simulink model "Buck_PI_DIGITAL_MG"  (R2024a)
settings: Solver=VariableStepAuto  StartTime=0.0  StopTime=0.1  RelTol=1e-3
libraries: spsSeriesRLCBranchLib x6, spsMeanLib x6, spsCurrentMeasurementLib x3, spsVoltageMeasurementLib x3, spsDiodeLib x2, spsDCVoltageSourceLib x2, spsMosfetLib x2, spsPWMGeneratorDCDCLib x2, sps_lib x1
settings Model: Creator=hardy  LastModifiedBy=marco
settings SolverCC: AlgebraicLoopSolver=TrustRegion
settings DebuggingCC: UnconnectedInputMsg=warning  UnconnectedOutputMsg=warning  UnconnectedLineMsg=warning
settings ModelReferenceCC: EnableRefExpFcnMdlSchedulingChecks=on
settings RTWCC: GPUComputeCapability=3.5

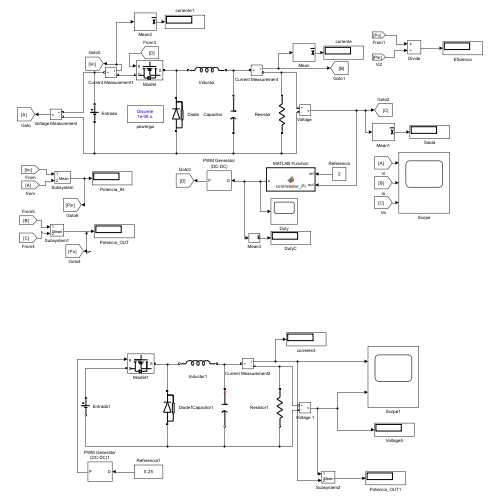
[thumbnail: Simulink's stored preview of the top-level diagram]
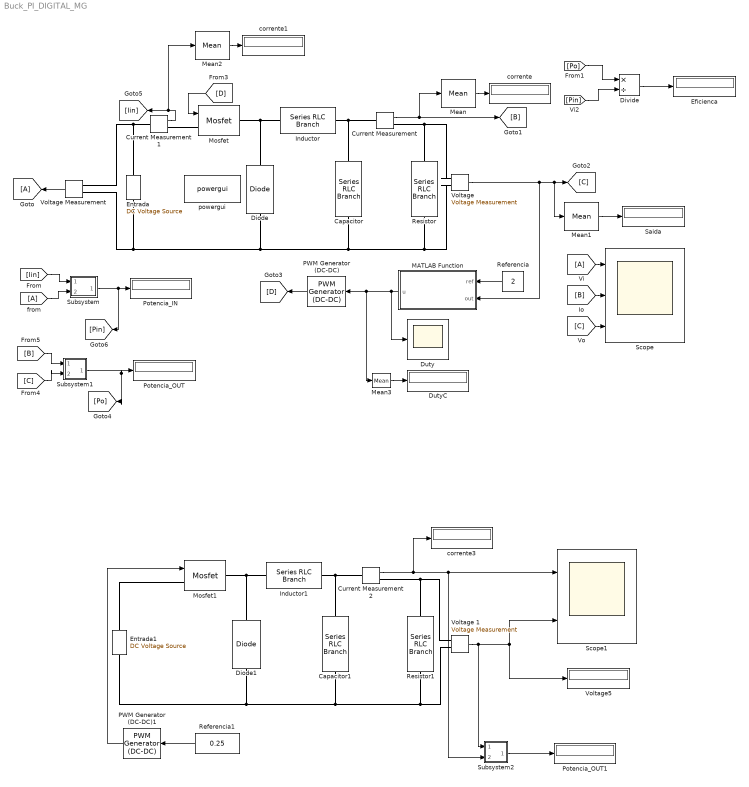
== system Buck_PI_DIGITAL_MG ==
  Capacitor : spsSeriesRLCBranchLib/Series RLC Branch  LConnTagsString=__new0  RConnTagsString=__new0  BranchType=C  Resistance=1  Inductance=1e-3  SetiL0=off  InitialCurrent=0  Capacitance=150e-6  Setx0=off  InitialVoltage=0  Measurements=None
  Capacitor1 : spsSeriesRLCBranchLib/Series RLC Branch  LConnTagsString=__new0  RConnTagsString=__new0  BranchType=C  Resistance=1  Inductance=1e-3  SetiL0=off  InitialCurrent=0  Capacitance=150e-6  Setx0=off  InitialVoltage=0  Measurements=None
  Current Measurement : spsCurrentMeasurementLib/Current Measurement  PhasorSimulation=off  OutputType=Complex  PSBequivalent=0
  Current Measurement1 : spsCurrentMeasurementLib/Current Measurement  PhasorSimulation=off  OutputType=Complex  PSBequivalent=0
  Current Measurement2 : spsCurrentMeasurementLib/Current Measurement  PhasorSimulation=off  OutputType=Complex  PSBequivalent=0
  Diode : spsDiodeLib/Diode  Ron=0.001  Lon=0  Vf=0  IC=0  UseSnubber=0  Rs=500  Cs=250e-9  Measurements=off
  Diode1 : spsDiodeLib/Diode  Ron=0.001  Lon=0  Vf=0  IC=0  UseSnubber=0  Rs=500  Cs=250e-9  Measurements=off
  Divide : Product  Inputs=*/
  Duty : Scope
  DutyC : Display
  Eficienca : Display
  Entrada : spsDCVoltageSourceLib/DC Voltage Source  Amplitude=10  Measurements=None
  Entrada1 : spsDCVoltageSourceLib/DC Voltage Source  Amplitude=10  Measurements=None
  Goto : Goto
  Inductor : spsSeriesRLCBranchLib/Series RLC Branch  LConnTagsString=__new0  RConnTagsString=__new0  BranchType=L  Resistance=1  Inductance=470e-6  SetiL0=off  InitialCurrent=0  Capacitance=1e-6  Setx0=off  InitialVoltage=0  Measurements=None
  Inductor1 : spsSeriesRLCBranchLib/Series RLC Branch  LConnTagsString=__new0  RConnTagsString=__new0  BranchType=L  Resistance=1  Inductance=470e-6  SetiL0=off  InitialCurrent=0  Capacitance=1e-6  Setx0=off  InitialVoltage=0  Measurements=None
  MATLAB Function : MATLAB Function  TreatAsAtomicUnit=on
  Mean{,1..3} (4 alike) : spsMeanLib/Mean  Freq=60  Vinit=0  Ts=0
  Mosfet : spsMosfetLib/Mosfet  Ron=0.1  Lon=0  Rd=0.01  Vfd=0  IC=0  Rs=1e5  Cs=inf  Measurements=off
  Mosfet1 : spsMosfetLib/Mosfet  Ron=0.1  Lon=0  Rd=0.01  Vfd=0  IC=0  Rs=1e5  Cs=inf  Measurements=off
  PWM Generator (DC-DC) : spsPWMGeneratorDCDCLib/PWM Generator (DC-DC)  Fsw=60000  Ts=1e-6
  PWM Generator (DC-DC)1 : spsPWMGeneratorDCDCLib/PWM Generator (DC-DC)  Fsw=60000  Ts=1e-6
  Potencia_IN : Display
  Potencia_OUT : Display
  Potencia_OUT1 : Display
  Referencia : Constant  Value=2
  Referencia1 : Constant  Value=0.25
  Resistor : spsSeriesRLCBranchLib/Series RLC Branch  LConnTagsString=__new0  RConnTagsString=__new0  BranchType=R  Resistance=1  Inductance=1e-3  SetiL0=off  InitialCurrent=0  Capacitance=1e-6  Setx0=off  InitialVoltage=0  Measurements=None
  Resistor1 : spsSeriesRLCBranchLib/Series RLC Branch  LConnTagsString=__new0  RConnTagsString=__new0  BranchType=R  Resistance=1  Inductance=1e-3  SetiL0=off  InitialCurrent=0  Capacitance=1e-6  Setx0=off  InitialVoltage=0  Measurements=None
  Saida : Display
  Scope : Scope  NumInputPorts=3
  Scope1 : Scope  NumInputPorts=2
  Subsystem : Subsystem
  Subsystem1 : Subsystem
  Subsystem2 : Subsystem
  Vi : From
  "Voltage " : spsVoltageMeasurementLib/Voltage Measurement  PhasorSimulation=off  OutputType=Complex  PSBequivalent=0
  Voltage 1 : spsVoltageMeasurementLib/Voltage Measurement  PhasorSimulation=off  OutputType=Complex  PSBequivalent=0
  Voltage Measurement : spsVoltageMeasurementLib/Voltage Measurement  PhasorSimulation=off  OutputType=Complex  PSBequivalent=0
  Voltage5 : Display
  corrente : Display
  corrente1 : Display
  corrente3 : Display
  from : From
  powergui : sps_lib/powergui  Priority=1  SimulationMode=Discrete  SampleTime=1e-6  frequency=60  Iterations=50  frequencyindice=0  Pbase=100e6  ErrMax=1e-4  UnitsV=kV  UnitsW=MW  buscounter=0  FunctionMessages=off  echomessages=off  EnableUseOfTLC=off  CurrentSourceSwitches=off  DisableSnubberDevices=off  DisableRonSwitches=off  DisableVfSwitches=off  DisplayEquations=off  AutomaticDiscreteSolvers=off  SolverType=Tustin/Backward Euler (TBE)  Interpol=off  ExternalGateDelay=off  methode=off  Ts=100  x0status=blocks  SPID=on  SwTol=0  HookPort=off  NonlinearTolerance=1e-4  nMaxIteration=100  ContinueOnMaxIteration=off  RestoreLinks=warning  ResistiveCurrentMeasurement=off  Frange=[0:2:500]  Ylog=off  Xlog=on  ShowGrid=off  save=off  variable=ZData  structure=0  ZoomFFT=off  StartTime=0.0  cycles=1  DisplayStyle=1  fundamental=60  FreqAxis=off  MaxFrequency=1000  frequencyindicesteady=1  RmsSteady=1  display=off
  wires:
  Voltage Measurement/1 -> Goto/1
  "Voltage "/1 -> MATLAB Function/2(out), Mean1/1, [C]
  Vi/1 -> Scope/1
  [B] -> Scope/2
  [C] -> Scope/3
  Current Measurement/1 -> [B], Mean/1
  Referencia/1 -> MATLAB Function/1(ref)
  PWM Generator (DC-DC)/1 -> [D]
  [D] -> Mosfet/1
  MATLAB Function/1(u) -> PWM Generator (DC-DC)/1, Mean3/1, Duty/1
  Mean/1 -> corrente/1
  Mean1/1 -> Saida/1
  Mean3/1 -> DutyC/1
  Divide/1 -> Eficienca/1
  [Pin] -> Divide/2
  [Po] -> Divide/1
  Subsystem/1(Mean) -> Potencia_IN/1, [Pin]
  [Iin] -> Subsystem/1(In1)
  from/1 -> Subsystem/2(In2)
  Subsystem1/1(Mean) -> Potencia_OUT/1, [Po]
  [B] -> Subsystem1/1(In1)
  [C] -> Subsystem1/2(In2)
  Mean2/1 -> corrente1/1
  Current Measurement1/1 -> Mean2/1, [Iin]
  Current Measurement2/1 -> Subsystem2/2(In2), Scope1/1, corrente3/1
  Referencia1/1 -> PWM Generator (DC-DC)1/1
  PWM Generator (DC-DC)1/1 -> Mosfet1/1
  Voltage 1/1 -> Subsystem2/1(In1), Voltage5/1, Scope1/2
  Subsystem2/1(Mean) -> Potencia_OUT1/1
  connections:
  Current Measurement1/LConn1 -- Entrada/RConn1 -- Voltage Measurement/LConn1
  Mosfet/RConn1 -- Inductor/LConn1 -- Diode/RConn1
  Capacitor/LConn1 -- Current Measurement/LConn1 -- Inductor/RConn1
  Resistor/LConn1 -- "Voltage "/LConn1 -- Current Measurement/RConn1
  Resistor/RConn1 -- Diode/LConn1 -- Entrada/LConn1 -- Voltage Measurement/LConn2 -- Capacitor/RConn1 -- "Voltage "/LConn2
  Current Measurement1/RConn1 -- Mosfet/LConn1
  Inductor1/LConn1 -- Diode1/RConn1 -- Mosfet1/RConn1
  Current Measurement2/LConn1 -- Inductor1/RConn1 -- Capacitor1/LConn1
  Resistor1/LConn1 -- Voltage 1/LConn1 -- Current Measurement2/RConn1
  Entrada1/LConn1 -- Diode1/LConn1 -- Voltage 1/LConn2 -- Resistor1/RConn1 -- Capacitor1/RConn1
  Entrada1/RConn1 -- Mosfet1/LConn1

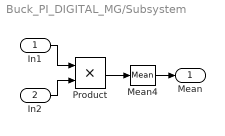
== system Buck_PI_DIGITAL_MG/Subsystem ==
  In1 : Inport
  In2 : Inport  Port=2
  Mean4 : spsMeanLib/Mean  Freq=60  Vinit=0  Ts=0
  Product : Product
  Mean : Outport
  wires:
  Product/1 -> Mean4/1
  In1/1 -> Product/1
  In2/1 -> Product/2
  Mean4/1 -> Mean/1

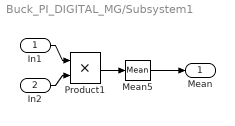
== system Buck_PI_DIGITAL_MG/Subsystem1 ==
  In1 : Inport
  In2 : Inport  Port=2
  Mean5 : spsMeanLib/Mean  Freq=60  Vinit=0  Ts=0
  Product1 : Product
  Mean : Outport
  wires:
  Product1/1 -> Mean5/1
  Mean5/1 -> Mean/1
  In1/1 -> Product1/1
  In2/1 -> Product1/2

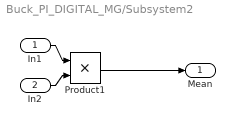
== system Buck_PI_DIGITAL_MG/Subsystem2 ==
  In1 : Inport
  In2 : Inport  Port=2
  Product1 : Product
  Mean : Outport
  wires:
  In2/1 -> Product1/2
  In1/1 -> Product1/1
  Product1/1 -> Mean/1

== matlab function Buck_PI_DIGITAL_MG/MATLAB Function ==
  data: ref input; u output; out input
function u = controlador_PI(ref, out)


Kp = 0.01;       % Ganho proporcional
Ki = 10;       % Ganho integral

% Persistência das variáveis
persistent integralErro
if isempty(integralErro)
    integralErro = 0;
end

% Cálculo do erro
erro = ref - out;

% Tempo de amostragem (ajuste conforme o sistema)
Ts = 1e-6;

% Integração do erro
integralErro = integralErro + erro * Ts;

% Saída do controlador
u = Kp * erro + Ki * integralErro;
